simulink library "lib_Timer_Counter"  (Simulink 8.2)
settings: Solver=ode45  StartTime=0.0  StopTime=10.0  RelTol=1e-3
settings Model: Creator=sunnyb  LastModifiedBy=sunnyb

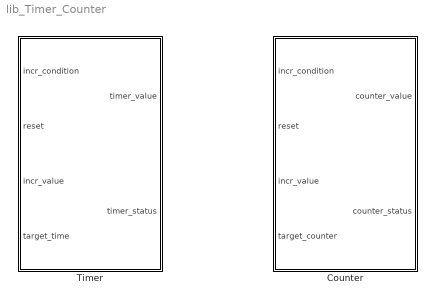
== system lib_Timer_Counter ==
  Counter : Subsystem
  Timer : Subsystem

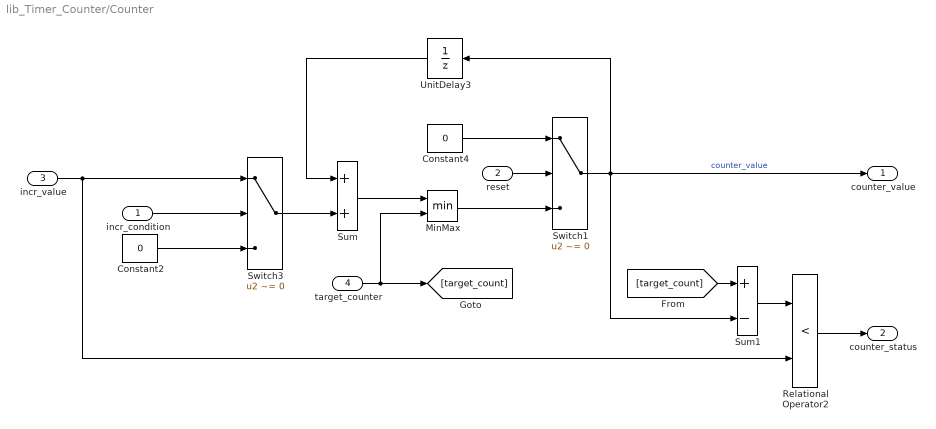
== system lib_Timer_Counter/Counter ==
  incr_condition : Inport
  reset : Inport  Port=2
  incr_value : Inport  Port=3
  target_counter : Inport  Port=4
  Constant2 : Constant  Value=0  OutDataTypeStr=Inherit: Inherit via back propagation
  Constant4 : Constant  Value=0  OutDataTypeStr=Inherit: Inherit via back propagation
  MinMax : MinMax  Inputs=2
  Relational Operator2 : RelationalOperator  Operator=<  OutDataTypeStr=boolean
  Sum : Sum
  Sum1 : Sum  Inputs=+-
  Switch1 : Switch  Criteria=u2 ~= 0  InputSameDT=on
  Switch3 : Switch  Criteria=u2 ~= 0  InputSameDT=on
  UnitDelay3 : UnitDelay  SampleTime=-1
      settings: AttributesFormatString=|
      | Initial = %<X0>
      | tsample = %<SampleTime>
  counter_value : Outport
  counter_status : Outport  Port=2
  wires:
  MinMax/1 -> Switch1/3
  Sum/1 -> MinMax/1
  Relational Operator2/1 -> counter_status/1
  incr_condition/1 -> Switch3/2
  target_counter/1 -> [target_count], MinMax/2
  [target_count] -> Sum1/1
  Sum1/1 -> Relational Operator2/1
  Constant2/1 -> Switch3/3
  incr_value/1 -> Switch3/1, Relational Operator2/2
  Switch3/1 -> Sum/2
  UnitDelay3/1 -> Sum/1
  reset/1 -> Switch1/2
  Constant4/1 -> Switch1/1
  Switch1/1 -> counter_value/1, Sum1/2, UnitDelay3/1  "counter_value"

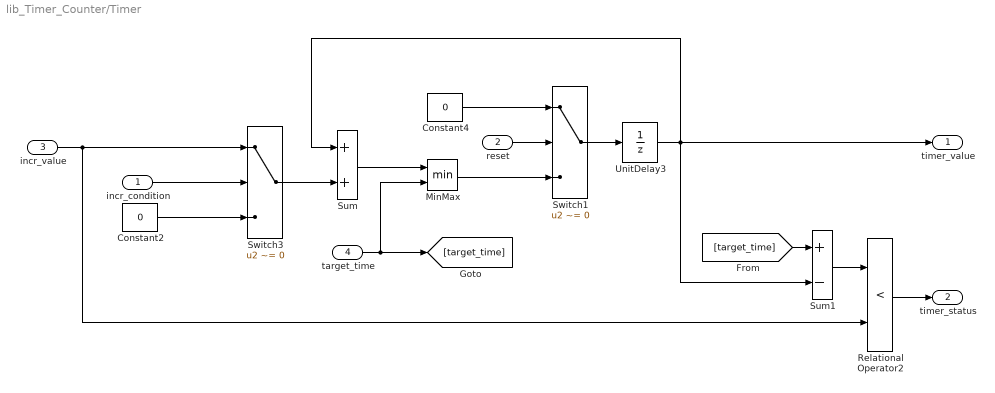
== system lib_Timer_Counter/Timer ==
  incr_condition : Inport
  reset : Inport  Port=2
  incr_value : Inport  Port=3
  target_time : Inport  Port=4
  Constant2 : Constant  Value=0  OutDataTypeStr=Inherit: Inherit via back propagation
  Constant4 : Constant  Value=0  OutDataTypeStr=Inherit: Inherit via back propagation
  MinMax : MinMax  Inputs=2
  Relational Operator2 : RelationalOperator  Operator=<  OutDataTypeStr=boolean
  Sum : Sum
  Sum1 : Sum  Inputs=+-
  Switch1 : Switch  Criteria=u2 ~= 0  InputSameDT=on
  Switch3 : Switch  Criteria=u2 ~= 0  InputSameDT=on
  UnitDelay3 : UnitDelay  SampleTime=-1
      settings: AttributesFormatString=|
      | Initial = %<X0>
      | tsample = %<SampleTime>
  timer_value : Outport
  timer_status : Outport  Port=2
  wires:
  Constant4/1 -> Switch1/1
  reset/1 -> Switch1/2
  Switch3/1 -> Sum/2
  incr_value/1 -> Relational Operator2/2, Switch3/1
  Constant2/1 -> Switch3/3
  Sum1/1 -> Relational Operator2/1
  [target_time] -> Sum1/1
  target_time/1 -> MinMax/2, [target_time]
  incr_condition/1 -> Switch3/2
  Relational Operator2/1 -> timer_status/1
  Sum/1 -> MinMax/1
  MinMax/1 -> Switch1/3
  Switch1/1 -> UnitDelay3/1
  UnitDelay3/1 -> Sum1/2, timer_value/1, Sum/1
